simulink model "planarBicopterGraduate"  (R2019b)
settings: Solver=ode1  StartTime=0.0  StopTime=100  FixedStep=0.001  RelTol=1e-3
PreLoadFcn:
  | clear P Pstruct
  | PStruct=Simulink.Bus
  | P(1,1)=Simulink.BusElement
  | P(2,1)=Simulink.BusElement
  | P(3,1)=Simulink.BusElement
  | P(4,1)=Simulink.BusElement
  | P(5,1)=Simulink.BusElement
  | P(6,1)=Simulink.BusElement
  | P(7,1)=Simulink.BusElement
  | P(8,1)=Simulink.BusElement
  | P(9,1)=Simulink.BusElement
  | P(10,1)=Simulink.BusElement
  | P(11,1)=Simulink.BusElement
  | P(12,1)=Simulink.BusElement
  | P(13,1)=Simulink.BusElement
  | P(14,1)=Simulink.BusElement
  | P(15,1)=Simulink.BusElement
  | P(1,1).Name='M'
  | P(2,1).Name='mRotor'
  | P(3,1).Name='J'
  | P(4,1).Name='d'
  | P(5,1).Name='mu'
  | P(6,1).Name='g'
  | P(7,1).Name='noVar'
  | P(8,1).Name='distPercent'
  | P(9,1).Name='vWind'
  | P(10,1).Name='kf'
  | P(11,1).Name='kv'
  | P(12,1).Name='bm'
  | P(13,1).Name='Jm'
  | P(14,1).Name='vSat'
  | P(15,1).Name='x0'
  | P(15,1).Dimensions = [6,1];
  | PStruct.Elements=P
libraries: commchan3 x5, simulink x2
settings Model: Creator=rushik  LastModifiedBy=rushik
settings DataIOCC: SaveOutput=off  SignalLogging=off  DSMLogging=off  SaveTime=off  ReturnWorkspaceOutputs=off

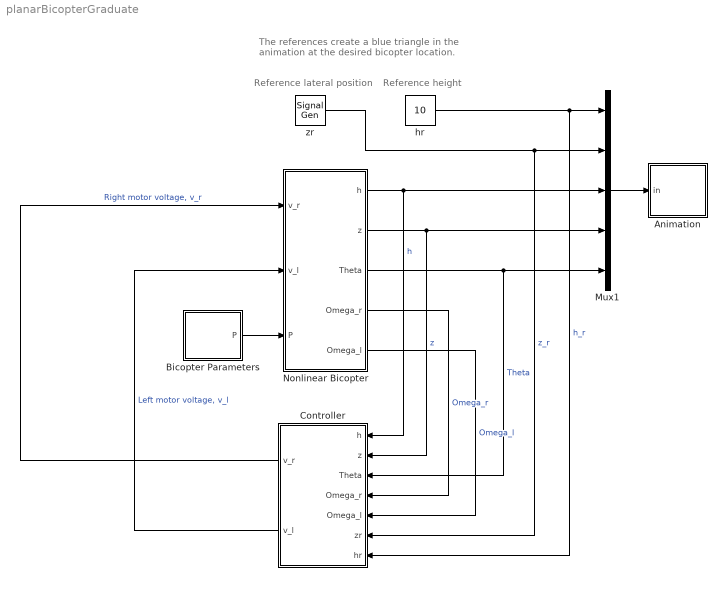
== system planarBicopterGraduate ==
  note: The references create a blue triangle in the
      | animation at the desired bicopter location.
  note: Reference height
  note: Reference lateral position
  Animation : Subsystem  mask(Pendulum plot){}
      mask help: Pendulum plot
      mask Help: Pendulum animation function using Handle graphics.
      mask Display: plot([-2 2],[10 10],[-2.5 -1.5],[10.5 10.5],[1.5 2.5],[10.5 10.5],0,0,0,20)
  Bicopter Parameters : Subsystem  mask{M=1, J=0.0042, d=0.3, mu=0.1, g=9.81, x0=[0;0;0;0;0;0], Value=10, Jm=0.004, bm=0.04, kv=12, kf=1.2e-6, mRotor=0.25, noVar=0, vWind=0, distPercent=0}
      mask prompts: M "Hub Mass"; J "Hub Inertia"; d "Arm Length"; mu "Momentum Drag Coefficient"; g "Gravity"; x0 "Initial State"; Value "Max Motor Voltage"; Jm "Motor Inertia"; bm "Damping Constant"; kv "Motor Voltage Constant"; kf "Propeller Thrust Constant"; mRotor "Motor Propeller Mass"; noVar "Noise Variance"; vWind "Wind Velocity"; distPercent "Parameter Variation Percentage"
      mask TypeOptions M: Constant1/Value
      mask TypeOptions J: Constant3/Value
      mask TypeOptions d: Constant4/Value
      mask TypeOptions mu: Constant5/Value
      mask TypeOptions g: Constant6/Value
      mask TypeOptions x0: Constant7/Value
      mask TypeOptions Value: Constant15/Value
      mask TypeOptions Jm: Constant14/Value
      mask TypeOptions bm: Constant13/Value
      mask TypeOptions kv: Constant12/Value
      mask TypeOptions kf: Constant11/Value
      mask TypeOptions mRotor: Constant2/Value
      mask TypeOptions noVar: Constant8/Value
      mask TypeOptions vWind: Constant10/Value
      mask TypeOptions distPercent: Constant9/Value
      mask DialogControl ParameterGroupVar Prompt: Bicopter
      mask DialogControl Container3 Prompt: Motor-Propeller Assembly
      mask DialogControl Container7 Prompt: Uncertainty and Noise
  Controller : Subsystem
  Mux1 : Mux  Inputs=5
  Nonlinear Bicopter : Subsystem
  hr : Constant  Value=10
  zr : SignalGenerator  WaveForm=square  Amplitude=1.5  Frequency=0.05
  wires:
  zr/1 -> Mux1/2, Controller/6(zr)  "z_r"
  Nonlinear Bicopter/1(h) -> Controller/1(h), Mux1/3  "h"
  Nonlinear Bicopter/2(z) -> Mux1/4, Controller/2(z)  "z"
  Nonlinear Bicopter/3(Theta) -> Mux1/5, Controller/3(Theta)  "Theta"
  Mux1/1 -> Animation/1(in)
  Bicopter Parameters/1(P) -> Nonlinear Bicopter/3(P)
  Controller/1(v_r) -> Nonlinear Bicopter/1(v_r)  "Right motor voltage, v_r"
  Controller/2(v_l) -> Nonlinear Bicopter/2(v_l)  "Left motor voltage, v_l"
  hr/1 -> Mux1/1, Controller/7(hr)  "h_r"
  Nonlinear Bicopter/4(Omega_r) -> Controller/4(Omega_r)  "Omega_r"
  Nonlinear Bicopter/5(Omega_l) -> Controller/5(Omega_l)  "Omega_l"

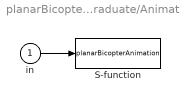
== system planarBicopterGraduate/Animation ==
  in : Inport
  S-function : S-Function  FunctionName=planarBicopterAnimation  SFunctionDeploymentMode=off  EnableBusSupport=off
      settings: DeleteFcn=pendan([],[],[],'DeleteBlock');
  wires:
  in/1 -> S-function/1

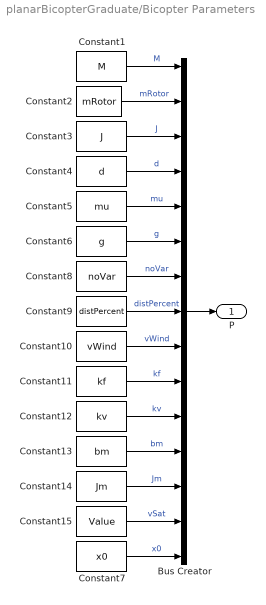
== system planarBicopterGraduate/Bicopter Parameters ==
  Bus Creator : BusCreator  Inputs=15  OutDataTypeStr=Bus: PStruct
  Constant1 : Constant  Value=M
  Constant10 : Constant  Value=vWind  VectorParams1D=off
  Constant11 : Constant  Value=kf  VectorParams1D=off
  Constant12 : Constant  Value=kv  VectorParams1D=off
  Constant13 : Constant  Value=bm  VectorParams1D=off
  Constant14 : Constant  Value=Jm  VectorParams1D=off
  Constant15 : Constant  Value=Value  VectorParams1D=off
  Constant2 : Constant  Value=mRotor
  Constant3 : Constant  Value=J
  Constant4 : Constant  Value=d
  Constant5 : Constant  Value=mu
  Constant6 : Constant  Value=g
  Constant7 : Constant  Value=x0  VectorParams1D=off
  Constant8 : Constant  Value=noVar  VectorParams1D=off
  Constant9 : Constant  Value=distPercent  VectorParams1D=off
  P : Outport
  wires:
  Bus Creator/1 -> P/1
  Constant7/1 -> Bus Creator/15  "x0"
  Constant5/1 -> Bus Creator/5  "mu"
  Constant3/1 -> Bus Creator/3  "J"
  Constant2/1 -> Bus Creator/2  "mRotor"
  Constant6/1 -> Bus Creator/6  "g"
  Constant4/1 -> Bus Creator/4  "d"
  Constant1/1 -> Bus Creator/1  "M"
  Constant8/1 -> Bus Creator/7  "noVar"
  Constant9/1 -> Bus Creator/8  "distPercent"
  Constant10/1 -> Bus Creator/9  "vWind"
  Constant11/1 -> Bus Creator/10  "kf"
  Constant12/1 -> Bus Creator/11  "kv"
  Constant13/1 -> Bus Creator/12  "bm"
  Constant14/1 -> Bus Creator/13  "Jm"
  Constant15/1 -> Bus Creator/14  "vSat"

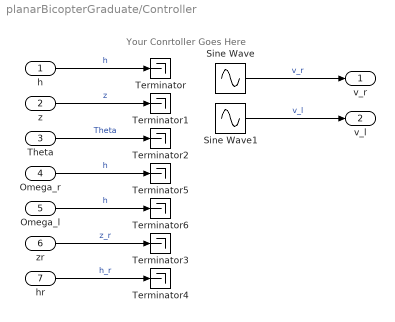
== system planarBicopterGraduate/Controller ==
  note: Your Conrtoller Goes Here
  h : Inport
  z : Inport  Port=2
  Theta : Inport  Port=3
  Omega_r : Inport  Port=4
  Omega_l : Inport  Port=5
  zr : Inport  Port=6
  hr : Inport  Port=7
  Sine Wave : Sin  Amplitude=0.002  Bias=8.3  SampleTime=0
  Sine Wave1 : Sin  Amplitude=0.002  Bias=8.3  Phase=0.1  SampleTime=0
  Terminator{,1..6} (7 alike) : Terminator
  v_r : Outport
  v_l : Outport  Port=2
  wires:
  Sine Wave/1 -> v_r/1  "v_r"
  Sine Wave1/1 -> v_l/1  "v_l"
  h/1 -> Terminator/1  "h"
  z/1 -> Terminator1/1  "z"
  Theta/1 -> Terminator2/1  "Theta"
  zr/1 -> Terminator3/1  "z_r"
  hr/1 -> Terminator4/1  "h_r"
  Omega_r/1 -> Terminator5/1  "h"
  Omega_l/1 -> Terminator6/1  "h"

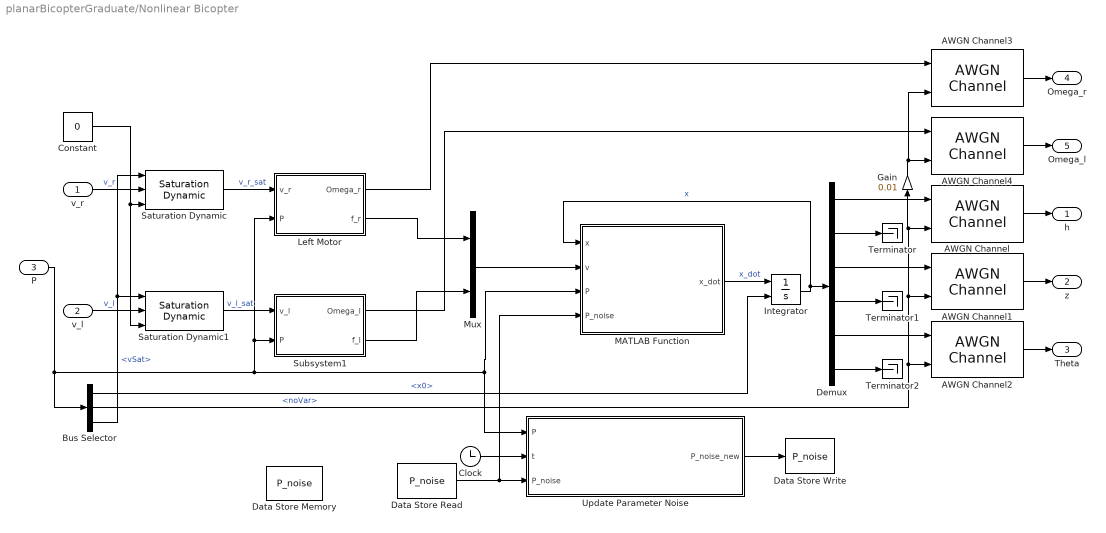
== system planarBicopterGraduate/Nonlinear Bicopter ==
  v_r : Inport
  v_l : Inport  Port=2
  P : Inport  Port=3
  AWGN Channel{,1..4} (5 alike) : commchan3/AWGN Channel  InputProcessing=Columns as channels (frame based)  seed=67  noiseMode=Variance from port  EbNodB=10  EsNodB=10  SNRdB=10  bitsPerSym=1  Ps=1  Tsym=1  variance=1
      settings: SourceProductName=Communications Toolbox
  Bus Selector : BusSelector  OutputSignals=x0,noVar,vSat
  Clock : Clock
  Constant : Constant  Value=0
  Data Store Memory : DataStoreMemory  DataStoreName=P_noise  ReadBeforeWriteMsg=warning  WriteAfterWriteMsg=warning  WriteAfterReadMsg=warning  InitialValue=[0;0;0;0;0;0;0;0]  ShowAdditionalParam=off  OutDataTypeStr=double
  Data Store Read : DataStoreRead  DataStoreName=P_noise
  Data Store Write : DataStoreWrite  DataStoreName=P_noise
  Demux : Demux  Outputs=6
  Gain : Gain  Gain=0.01
  Integrator : Integrator  InitialConditionSource=external
  Left Motor : Subsystem
  MATLAB Function : MATLAB Function  TreatAsAtomicUnit=on
  Mux : Mux  Inputs=2
  Saturation Dynamic : simulink/Discontinuities/Saturation Dynamic  OutMin=[]  OutMax=[]  OutDataTypeStr=Inherit: Same as second input  OutDataType=fixdt(1, 16)  OutScaling=2^-10  DoSatur=off
  Saturation Dynamic1 : simulink/Discontinuities/Saturation Dynamic  OutMin=[]  OutMax=[]  OutDataTypeStr=Inherit: Same as second input  OutDataType=fixdt(1, 16)  OutScaling=2^-10  DoSatur=off
  Subsystem1 : Subsystem
  Terminator : Terminator
  Terminator1 : Terminator
  Terminator2 : Terminator
  Update Parameter Noise : MATLAB Function  TreatAsAtomicUnit=on
  h : Outport
  z : Outport  Port=2
  Theta : Outport  Port=3
  Omega_r : Outport  Port=4
  Omega_l : Outport  Port=5
  wires:
  MATLAB Function/1(x_dot) -> Integrator/1  "x_dot"
  v_r/1 -> Saturation Dynamic/2  "v_r"
  Bus Selector/1 -> Integrator/2  "<x0>"
  P/1 -> Subsystem1/2(P), Left Motor/2(P), MATLAB Function/3(P), Update Parameter Noise/1(P), Bus Selector/1
  v_l/1 -> Saturation Dynamic1/2  "v_l"
  Demux/6 -> Terminator2/1
  Demux/2 -> Terminator/1
  Demux/4 -> Terminator1/1
  Integrator/1 -> MATLAB Function/1(x), Demux/1  "x"
  Bus Selector/2 -> AWGN Channel2/2, AWGN Channel1/2, AWGN Channel/2, Gain/1  "<noVar>"
  Demux/1 -> AWGN Channel/1
  Demux/3 -> AWGN Channel1/1
  Demux/5 -> AWGN Channel2/1
  AWGN Channel/1 -> h/1
  AWGN Channel1/1 -> z/1
  AWGN Channel2/1 -> Theta/1
  Update Parameter Noise/1(P_noise_new) -> Data Store Write/1
  Clock/1 -> Update Parameter Noise/2(t)
  Data Store Read/1 -> MATLAB Function/4(P_noise), Update Parameter Noise/3(P_noise)
  Mux/1 -> MATLAB Function/2(v)
  Saturation Dynamic/1 -> Left Motor/1(v_r)  "v_r_sat"
  Left Motor/2(f_r) -> Mux/1
  Saturation Dynamic1/1 -> Subsystem1/1(v_l)  "v_l_sat"
  Subsystem1/2(f_l) -> Mux/2
  Constant/1 -> Saturation Dynamic1/3, Saturation Dynamic/3
  Bus Selector/3 -> Saturation Dynamic1/1, Saturation Dynamic/1  "<vSat>"
  Left Motor/1(Omega_r) -> AWGN Channel3/1
  Subsystem1/1(Omega_l) -> AWGN Channel4/1
  AWGN Channel3/1 -> Omega_r/1
  AWGN Channel4/1 -> Omega_l/1
  Gain/1 -> AWGN Channel4/2, AWGN Channel3/2

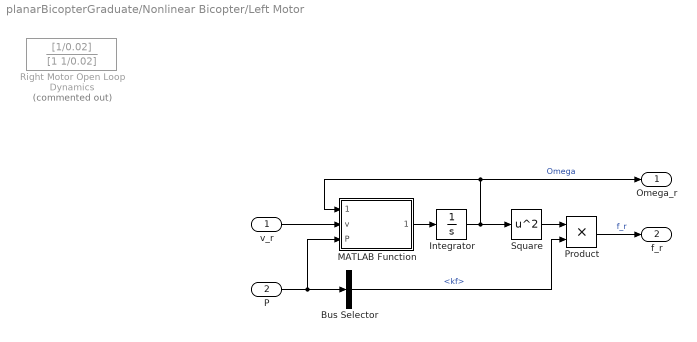
== system planarBicopterGraduate/Nonlinear Bicopter/Left Motor ==
  v_r : Inport
  P : Inport  Port=2
  Bus Selector : BusSelector  OutputSignals=kf
  Integrator : Integrator
  MATLAB Function : MATLAB Function  TreatAsAtomicUnit=on
  Product : Product
  Right Motor Open Loop Dynamics : TransferFcn  Commented=on  Numerator=[1/0.02]  Denominator=[1 1/0.02]
  Square : Math  Operator=square  SignedPower=off  SaturateOnIntegerOverflow=on
  Omega_r : Outport
  f_r : Outport  Port=2
  wires:
  v_r/1 -> MATLAB Function/2(v)
  P/1 -> MATLAB Function/3(P), Bus Selector/1
  MATLAB Function/1(OmegaDot) -> Integrator/1
  Integrator/1 -> Square/1, Omega_r/1, MATLAB Function/1(Omega)  "Omega"
  Square/1 -> Product/1
  Bus Selector/1 -> Product/2  "<kf>"
  Product/1 -> f_r/1  "f_r"

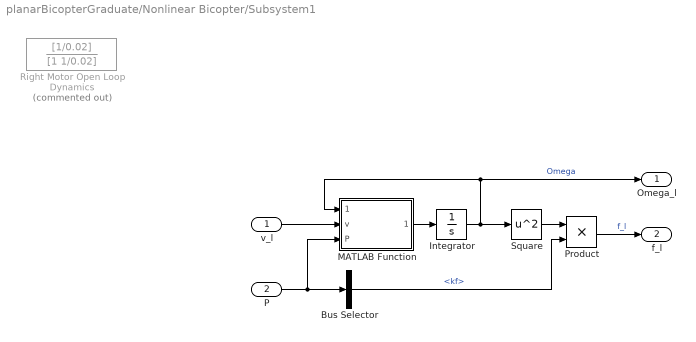
== system planarBicopterGraduate/Nonlinear Bicopter/Subsystem1 ==
  v_l : Inport
  P : Inport  Port=2
  Bus Selector : BusSelector  OutputSignals=kf
  Integrator : Integrator
  MATLAB Function : MATLAB Function  TreatAsAtomicUnit=on
  Product : Product
  Right Motor Open Loop Dynamics : TransferFcn  Commented=on  Numerator=[1/0.02]  Denominator=[1 1/0.02]
  Square : Math  Operator=square  SignedPower=off  SaturateOnIntegerOverflow=on
  Omega_l : Outport
  f_l : Outport  Port=2
  wires:
  v_l/1 -> MATLAB Function/2(v)
  P/1 -> MATLAB Function/3(P), Bus Selector/1
  MATLAB Function/1(OmegaDot) -> Integrator/1
  Integrator/1 -> Square/1, Omega_l/1, MATLAB Function/1(Omega)  "Omega"
  Square/1 -> Product/1
  Bus Selector/1 -> Product/2  "<kf>"
  Product/1 -> f_l/1  "f_l"

== matlab function planarBicopterGraduate/Nonlinear Bicopter/Subsystem1/MATLAB Function ==
  data: Omega input; v input; OmegaDot output; P input
function OmegaDot = fcn(Omega,v,P)
OmegaDot = -(P.bm/P.Jm)*Omega+(P.kv/P.Jm)*v;
end

== matlab function planarBicopterGraduate/Nonlinear Bicopter/Left Motor/MATLAB Function ==
  data: Omega input; v input; OmegaDot output; P input
function OmegaDot = fcn(Omega,v,P)
OmegaDot = -(P.bm/P.Jm)*Omega+(P.kv/P.Jm)*v;
end

== matlab function planarBicopterGraduate/Nonlinear Bicopter/MATLAB Function ==
  settings: updateMethod=DISCRETE
  data: x input; v input; x_dot output; P input; P_noise input

function x_dot = VTOLNonlinearDynamics(x,v,P, P_noise)

M = P.M + P_noise(1);
m = P.mRotor + P_noise(2);
J = P.J + P_noise(3);
d = P.d + P_noise(4);
mu = P.mu+ P_noise(5);
g = P.g + P_noise(6);
c_d = 1;
v_wind = P.vWind + P_noise(7);
theta_wind = P_noise(8);

F_drag_wind_vert = c_d*v_wind*sin(theta_wind);
F_drag_wind_horiz = c_d*v_wind*cos(theta_wind);

thrustToTorque = [1   1;
                  d  -d];

u = thrustToTorque*v;

h = x(1);
hD = x(2);
z = x(3);
zD = x(4);
T = x(5);
TD = x(6);

F = u(1);
tau = u(2);

x_dot = [hD;
         -g + (1/(M + 2*m)) * (cos(T) * F + F_drag_wind_vert);
         zD;
         (1/(M + 2*m)) * (-mu * zD - sin(T) * F + F_drag_wind_horiz);
         TD;
         (1/(2 * m * d^2 + J)) * tau];
     
end

== matlab function planarBicopterGraduate/Nonlinear Bicopter/Update Parameter Noise ==
  settings: updateMethod=DISCRETE
  data: P input; t input; P_noise_new output; P_noise input
function P_noise_new  = updateParameterNoise(P,t,P_noise)
if t<=0.001
    M = P.M ;
    m = P.mRotor ;
    J = P.J ;
    d = P.d ;
    mu = P.mu;
    g = P.g ;
    distPercent = P.distPercent;
    MNoise = (distPercent*M/100)*rand - distPercent*M/200;
    mNoise = (distPercent*m/100)*rand - distPercent*m/200;
    JNoise = (distPercent*J/100)*rand - distPercent*J/200;
    dNoise = (distPercent*d/100)*rand - distPercent*d/200;
    muNoise = (distPercent*mu/100)*rand - distPercent*mu/200;
    gNoise = (distPercent*g/100)*rand - distPercent*g/200;
    
    P_noise_new = ...
    [MNoise ;
     mNoise ;
     JNoise ;
     dNoise ;
    muNoise ;
     gNoise;
     P_noise(7);
     P_noise(8)];
elseif mod(round(t/0.002),1000)==0 %0.002 is the sample time
    vWind = P.vWind;
    vWindNoise = 20*vWind/100*rand - 20*vWind/200;
    thetaWindNoise = (0.5)*rand - 0.25;
    P_noise_new = ...
    [P_noise(1:6,1);
     vWindNoise;
     thetaWindNoise];
else
    P_noise_new = P_noise;
end
